simulink model "missileSystem"  (R2015a)
settings: Solver=ode45  StartTime=0.0  StopTime=10.0  RelTol=1e-3
values from neighbouring files (symbols this model uses):
  Arb = df(:,1:2)    [getRigidBodySS.m]
  Brb = df(:,end)    [getRigidBodySS.m]
  Crb = dg(:,1:2)    [getRigidBodySS.m]
  Drb = dg(:,end)    [getRigidBodySS.m]
  wAct = 2*pi*25    (= 157.079632679)    [initVibeSupp.m]
  zAct = 0.707    [initVibeSupp.m]
settings Model: CovSFcnEnable=off  Creator=s220385  LastModifiedBy=anatole
settings DebuggingCC: SolverPrmCheckMsg=warning

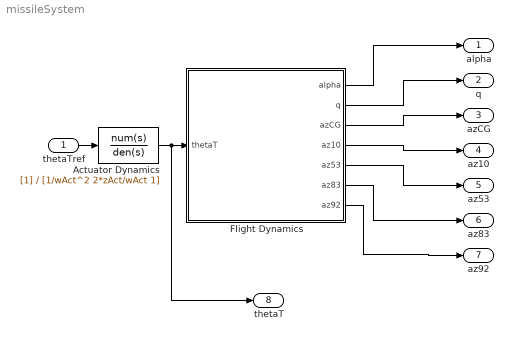
== system missileSystem ==
  thetaTref : Inport
  Actuator Dynamics : TransferFcn  Denominator=[1/wAct^2 2*zAct/wAct 1]
  Flight Dynamics : Subsystem  TreatAsAtomicUnit=on
      settings: MinAlgLoopOccurrences=on
      mask Display:
      | port_label('input', 1, '\theta_T','texmode','on')
      | 
      | port_label('output', 1, '\alpha','texmode','on')
      | port_label('output', 2, 'q','texmode','on')
      | port_label('output', 3, 'a_{zCG}','texmode','on')
      | port_label('output', 4, 'a_{z10}','texmode','on')
      | port_label('output', 5, 'a_{z53}','texmode','on')
      | port_label('output', 6, 'a_{z83}','texmode','on')
      | port_label('output', 7, 'a_{z91}','texmode','on')
  alpha : Outport
  q : Outport  Port=2
  azCG : Outport  Port=3
  az10 : Outport  Port=4
  az53 : Outport  Port=5
  az83 : Outport  Port=6
  az92 : Outport  Port=7
  "thetaT " : Outport  Port=8
  wires:
  Flight Dynamics/4(az10) -> az10/1
  Flight Dynamics/2(q) -> q/1
  Flight Dynamics/1(alpha) -> alpha/1
  thetaTref/1 -> Actuator Dynamics/1
  Flight Dynamics/3(azCG) -> azCG/1
  Flight Dynamics/5(az53) -> az53/1
  Flight Dynamics/6(az83) -> az83/1
  Flight Dynamics/7(az92) -> az92/1
  Actuator Dynamics/1 -> "thetaT "/1, Flight Dynamics/1(thetaT)

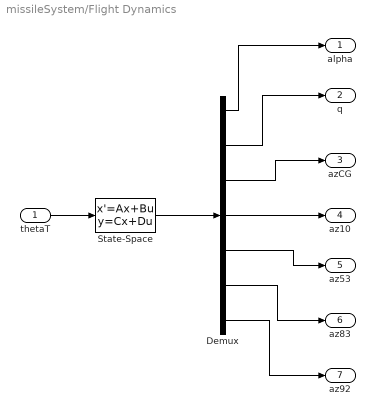
== system missileSystem/Flight Dynamics ==
  thetaT : Inport
  Demux : Demux  Outputs=7
  State-Space : StateSpace  A=Arb  B=Brb  C=Crb  D=Drb  X0=0
  alpha : Outport
  q : Outport  Port=2
  azCG : Outport  Port=3
  az10 : Outport  Port=4
  az53 : Outport  Port=5
  az83 : Outport  Port=6
  az92 : Outport  Port=7
  wires:
  thetaT/1 -> State-Space/1
  State-Space/1 -> Demux/1
  Demux/3 -> azCG/1
  Demux/2 -> q/1
  Demux/4 -> az10/1
  Demux/1 -> alpha/1
  Demux/5 -> az53/1
  Demux/6 -> az83/1
  Demux/7 -> az92/1
